simulink model "Zad_2_1_test"  (Simulink 10.0)
settings: Solver=FixedStepDiscrete  StartTime=0.0  StopTime=Tend  FixedStep=Tp  RelTol=1e-3  EnableMultiTasking=on
values from neighbouring files (symbols this model uses):
  c1o = 0.99    [ZADANIE_1_2.m]    (also in ZADANIE_2_1.m = 0; Zad_1_1.m = 0; Zad_1_1_8_kolorowe.m; Zad_2_1_zapominanie.m = 0)
  Td = 1500    [ZADANIE_1_2.m]    (also in ZADANIE_2_1.m = 500; Zad_1_1.m; Zad_1_1_8_kolorowe.m; Zad_2_1_zapominanie.m = 500)
  Tp = 0.1    [ZADANIE_1_2.m]    (also in ZADANIE_2_1.m; Zad_1_1.m; Zad_1_1_8_kolorowe.m; Zad_2_1_zapominanie.m)
libraries: simulink x2
settings Model: Creator=mgmil  LastModifiedBy=mgmil
settings DataIOCC: LimitDataPoints=on  SignalLoggingSaveFormat=ModelDataLogs
settings OptimizationCC: InitFltsAndDblsToZero=on
settings DebuggingCC: SaveWithParameterizedLinksMsg=none  SignalResolutionControl=TryResolveAllWithWarning  SolverPrmCheckMsg=warning  MultiTaskDSMMsg=warning  MultiTaskCondExecSysMsg=none  FcnCallInpInsideContextMsg=warning
settings SFSimCC: SimUseLocalCustomCode=on  CustomCodeUndefinedFunction=FilterOut
settings RTWCC: RTWUseLocalCustomCode=on
settings GRTTargetCC: TargetFcnLib=ansi_tfl_tmw.mat

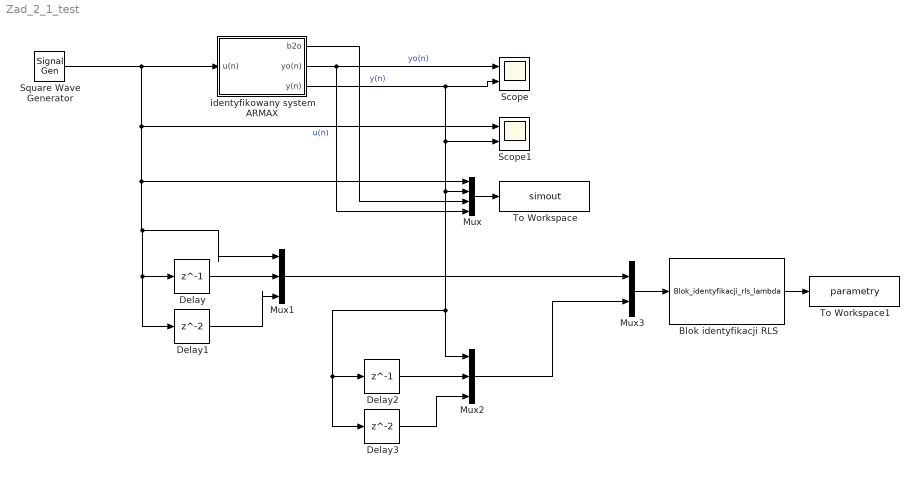
== system Zad_2_1_test ==
  Blok identyfikacji RLS : MATLABFcn  MATLABFcn=Blok_identyfikacji_rls_lambda
  Delay : Delay  DelayLength=1
  Delay1 : Delay
  Delay2 : Delay  DelayLength=1
  Delay3 : Delay
  Mux : Mux
  Mux1 : Mux  Inputs=3
  Mux2 : Mux  Inputs=3
  Mux3 : Mux  Inputs=2
  Scope : Scope  NumInputPorts=2
  Scope1 : Scope  NumInputPorts=2
  Square Wave Generator : SignalGenerator  WaveForm=square  Frequency=0.025
  To Workspace : ToWorkspace  VariableName=simout  SampleTime=-1
  To Workspace1 : ToWorkspace  VariableName=parametry  SampleTime=-1
  identyfikowany system ARMAX : Subsystem
  wires:
  Square Wave Generator/1 -> Scope1/1, Delay1/1, Delay/1, Mux1/1, Mux/1, identyfikowany system ARMAX/1(u(n))  "u(n)"
  identyfikowany system ARMAX/2(yo(n)) -> Mux/4, Scope/1  "yo(n)"
  identyfikowany system ARMAX/3(y(n)) -> Scope/2, Scope1/2, Mux2/1, Delay2/1, Delay3/1, Mux/2  "y(n)"
  Mux/1 -> To Workspace/1
  identyfikowany system ARMAX/1(b2o) -> Mux/3
  Mux1/1 -> Mux3/1
  Delay/1 -> Mux1/2
  Delay1/1 -> Mux1/3
  Delay2/1 -> Mux2/2
  Delay3/1 -> Mux2/3
  Mux2/1 -> Mux3/2
  Mux3/1 -> Blok identyfikacji RLS/1
  Blok identyfikacji RLS/1 -> To Workspace1/1

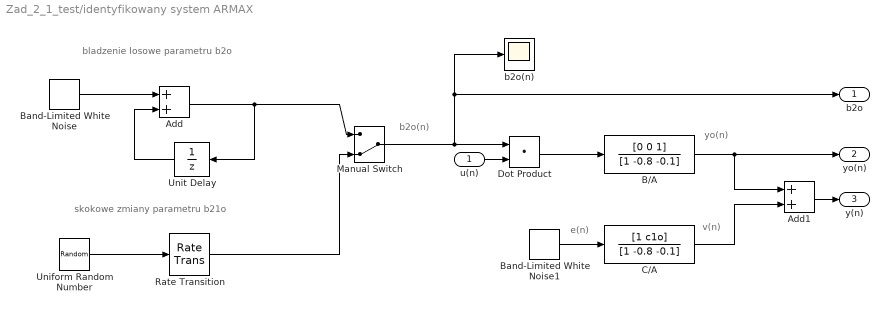
== system Zad_2_1_test/identyfikowany system ARMAX ==
  note: e(n)
  note: v(n)
  note: yo(n)
  note: b2o(n)
  note: skokowe zmiany parametru b21o
  note: bladzenie losowe parametru b2o
  u(n) : Inport
  Add : Sum
  Add1 : Sum
  B/A : DiscreteFilter  Numerator=[0 0 1]  Denominator=[1 -0.8 -0.1]  SampleTime=Tp
  Band-Limited White Noise : simulink/Sources/Band-Limited White Noise  Cov=[0.00001*Tp]  Ts=Tp  seed=[23341]
  Band-Limited White Noise1 : simulink/Sources/Band-Limited White Noise  Cov=[0.001*Tp]  Ts=Tp  seed=[23341]
  C/A : DiscreteFilter  Numerator=[1 c1o]  Denominator=[1 -0.8 -0.1]  SampleTime=Tp
  Dot Product : DotProduct  InputSameDT=on  OutDataTypeStr=Inherit: Inherit via internal rule
  Manual Switch : ManualSwitch  CurrentSetting=0
  Rate Transition : RateTransition  InitialCondition=0.5  OutPortSampleTime=Tp
  Uniform Random Number : UniformRandomNumber  Minimum=0.1  Maximum=0.8  Seed=2  SampleTime=Td
  Unit Delay : UnitDelay  SampleTime=Tp
  b2o(n) : Scope
  b2o : Outport
  yo(n) : Outport  Port=2
  y(n) : Outport  Port=3
  wires:
  Band-Limited White Noise/1 -> Add/1
  Add/1 -> Unit Delay/1, Manual Switch/1
  Unit Delay/1 -> Add/2
  Uniform Random Number/1 -> Rate Transition/1
  Rate Transition/1 -> Manual Switch/2
  Manual Switch/1 -> Dot Product/1, b2o/1, b2o(n)/1
  Dot Product/1 -> B/A/1
  C/A/1 -> Add1/2
  B/A/1 -> Add1/1, yo(n)/1
  Band-Limited White Noise1/1 -> C/A/1
  u(n)/1 -> Dot Product/2
  Add1/1 -> y(n)/1
